simulink library "SendToInputDevice"  (R2016b)
settings: Solver=VariableStepAuto  StartTime=0.0  StopTime=10.0  RelTol=1e-3
libraries: xpcethercatlib x2
settings Model: Creator=Nathan  LastModifiedBy=march

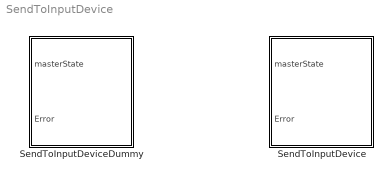
== system SendToInputDevice ==
  SendToInputDevice : Subsystem
  "SendToInputDeviceDummy " : Subsystem

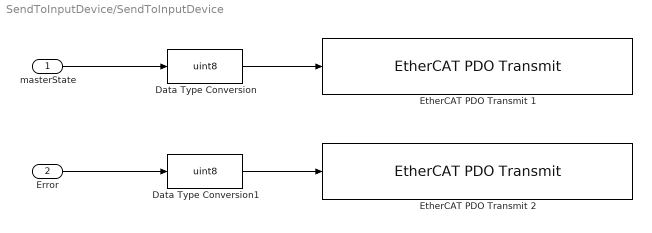
== system SendToInputDevice/SendToInputDevice ==
  masterState : Inport
  Error : Inport  Port=2
  Data Type Conversion : DataTypeConversion  OutDataTypeStr=uint8  RndMeth=Nearest
  Data Type Conversion1 : DataTypeConversion  OutDataTypeStr=uint8  RndMeth=Nearest
  EtherCAT PDO Transmit 1 : xpcethercatlib/EtherCAT PDO Transmit   Priority=3  sig_name=InputDevice.Outputs.actualStateMarch  sig_offset=720  sig_type=uint8  type_size=8  sig_dim=1  device_id=0  sample_time=0.002000
  EtherCAT PDO Transmit 2 : xpcethercatlib/EtherCAT PDO Transmit   Priority=3  sig_name=InputDevice.Outputs.masterError  sig_offset=728  sig_type=uint8  type_size=8  sig_dim=1  device_id=0  sample_time=0.002000
  wires:
  Data Type Conversion1/1 -> EtherCAT PDO Transmit 2/1
  Data Type Conversion/1 -> EtherCAT PDO Transmit 1/1
  Error/1 -> Data Type Conversion1/1
  masterState/1 -> Data Type Conversion/1

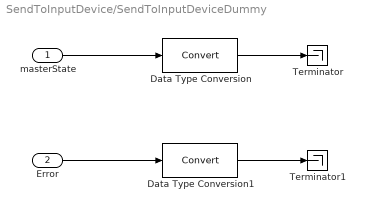
== system SendToInputDevice/SendToInputDeviceDummy  ==
  masterState : Inport
  Error : Inport  Port=2
  Data Type Conversion : DataTypeConversion
  Data Type Conversion1 : DataTypeConversion
  Terminator : Terminator
  Terminator1 : Terminator
  wires:
  Data Type Conversion1/1 -> Terminator1/1
  Data Type Conversion/1 -> Terminator/1
  Error/1 -> Data Type Conversion1/1
  masterState/1 -> Data Type Conversion/1
